simulink model "traffic_blind_test"  (Simulink 8.7)
settings: Solver=FixedStepAuto  StartTime=0.0  StopTime=75  FixedStep=0.01  RelTol=1e-3
settings Model: Creator=eispin  LastModifiedBy=eispin
settings DataIOCC: LimitDataPoints=off  SaveFormat=Dataset
settings DebuggingCC: UnderspecifiedInitializationDetection=Simplified  MergeDetectMultiDrivingBlocksExec=error
settings HardwareCC: ProdBitPerPointer=64  ProdLargestAtomicFloat=Float  ProdIntDivRoundTo=Zero  ProdEndianess=LittleEndian  ProdWordSize=64  ProdHWDeviceType=Intel->x86-64 (Windows64)
settings ModelReferenceCC: PropagateSignalLabelsOutOfModel=on
settings ConfigComp: CovModelRefEnable=off

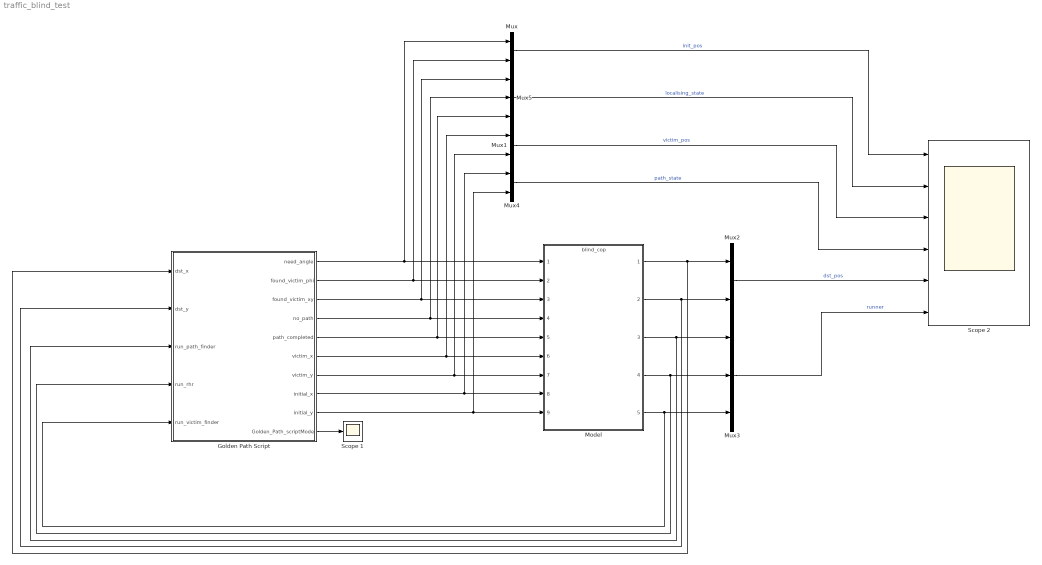
== system traffic_blind_test ==
  Golden Path Script : Stateflow chart  TreatAsAtomicUnit=on
  Model : ModelReference  ModelNameDialog=blind_cop  SimulationMode=Normal  ModelReferenceVersion=1.102
  Mux{,1..2,4} (4 alike) : Mux  Inputs=2
  Mux3 : Mux  Inputs=3
  Mux5 : Mux  Inputs=3
  Scope 1 : Scope
  Scope 2 : Scope  NumInputPorts=6
  wires:
  Model/1 -> Golden Path Script/1(dst_x), Mux2/1
  Model/2 -> Mux2/2, Golden Path Script/2(dst_y)
  Model/3 -> Mux3/1, Golden Path Script/3(run_path_finder)
  Model/4 -> Mux3/2, Golden Path Script/4(run_rhr)
  Model/5 -> Mux3/3, Golden Path Script/5(run_victim_finder)
  Mux3/1 -> Scope 2/6  "runner"
  Mux2/1 -> Scope 2/5  "dst_pos"
  Mux4/1 -> Scope 2/4  "path_state"
  Mux1/1 -> Scope 2/3  "victim_pos"
  Mux5/1 -> Scope 2/2  "localising_state"
  Mux/1 -> Scope 2/1  "init_pos"
  Golden Path Script/1(need_angle) -> Model/1, Mux/1
  Golden Path Script/2(found_victim_phi) -> Model/2, Mux/2
  Golden Path Script/4(no_path) -> Model/4, Mux5/2
  Golden Path Script/3(found_victim_xy) -> Model/3, Mux5/1
  Golden Path Script/6(victim_x) -> Model/6, Mux1/1
  Golden Path Script/5(path_completed) -> Mux5/3, Model/5
  Golden Path Script/7(victim_y) -> Model/7, Mux1/2
  Golden Path Script/8(initial_x) -> Model/8, Mux4/1
  Golden Path Script/9(initial_y) -> Model/9, Mux4/2
  Golden Path Script/10(Golden_Path_scriptMode) -> Scope 1/1

== stateflow chart Golden Path Script ==
  state Consistent
    state InitWait
      en:
      expect_dst_x = -1;
      expect_dst_y = -1;
      expect_run_path_finder = 0;
      expect_run_rhr = 1;
      expect_run_victim_finder = 0;
    state StartInterruptA
      en:
      need_angle = 1;
      expect_run_rhr = 0;
      expect_run_victim_finder = 1;
    state DoneInterruptA
      en:
      need_angle = 0;
    state DoneIsrA
      en:
      found_victim_phi = 1;
      expect_run_victim_finder = 0;
    state resumeAfterA
      en:
      found_victim_phi = 0;
      expect_run_rhr = 1;
    state StartInterruptB
      en:
      need_angle = 1;
      expect_run_rhr = 0;
      expect_run_victim_finder = 1;
    state DoneInterruptB
      en:
      found_victim_phi = 1;
      expect_run_victim_finder = 0;
    state DoneIsrB
      en:
      need_angle = 0;
    state resumeAfterB
      en:
      found_victim_phi = 0;
      expect_run_rhr = 1;
    state DoneIsrC
      en:
      found_victim_xy = 1;
      expect_run_victim_finder = 0;
      expect_run_path_finder = 1;
      expect_dst_x = victim_x;
      expect_dst_y = victim_y;
    state StartInterruptC
      en:
      need_angle = 1;
      expect_run_rhr = 0;
      expect_run_victim_finder = 1;
    state PathFailingA
      % Note that traffic cop should be
      % time-unaware here
      en:
      no_path = 1;
      expect_run_rhr = 1;
      expect_run_path_finder = 0;
    state RhrNearlyOverA
      en:
      expect_run_rhr = -1;
      expect_run_path_finder = -1;
    state RhrOverA
      en:
      % Still expect victim's coords!
      expect_run_rhr = 0;
      expect_run_path_finder = 1;
    state RhringA
      % Check that it doesn't depend on
      % no_path in a weird way
      en:
      no_path = 0;
    state DoneA
      en:
      path_completed = 1;
      expect_run_path_finder = 0;
    state DockingA
      % Waited to make sure that the traffic cop waits on us.
      en:
      path_completed = 0;
      expect_run_path_finder = -1;
      expect_dst_x = -1;
      expect_dst_y = -1;
    state ResumeAfterA
      en:
      expect_run_path_finder = 1;
      expect_dst_x = initial_x;
      expect_dst_y = initial_y;
    state RhrNearlyOverB
      en:
      expect_run_rhr = -1;
      expect_run_path_finder = -1;
    state RhringB
      % Check that it doesn't depend on
      % no_path in a weird way
      en:
      no_path = 0;
    state DoneB
      en:
      path_completed = 1;
      expect_run_path_finder = 0;
    state PathFailingb
      % Note that traffic cop should be
      % time-unaware here
      en:
      no_path = 1;
      expect_run_rhr = 1;
      expect_run_path_finder = 0;
    state RhrOverB
      en:
      % Still expect initial coords!
      expect_run_rhr = 0;
      expect_run_path_finder = 1;
    state TestReaction1
      en:
      path_completed = 0;
    state TestReaction2
      en:
      no_path = 1;
    state TestReaction3
      en:
      found_victim_xy = 1;
    state TestReaction4
      en:
      need_angle = 1;
    state TestReaction5
      en:
      found_victim_phi = 1;
    state TestReaction6
      en:
      path_completed = 1;
    state TestReaction7
      en:
      found_victim_xy = 1;
      initial_x = 12;
      initial_y = 11;
      victim_x = 10;
      victim_y = 9.01;
    state TestReaction8
      en:
      need_angle = 1;
    note: And then, try to confuse the traffic cop by sending random bullshit
        | (which it should ignore)
    (default) -> InitWait
    DoneIsrB -> resumeAfterB : [after(0.5,sec)]
    DoneIsrA -> resumeAfterA : [after(0.5,sec)]
    InitWait -> StartInterruptA : [after(0.5,sec)]
    resumeAfterA -> StartInterruptB : [after(0.5,sec)]
    resumeAfterB -> StartInterruptC : [after(0.5,sec)]
    StartInterruptA -> DoneInterruptA : [after(0.5,sec)]
    StartInterruptB -> DoneInterruptB : [after(0.5,sec)]
    StartInterruptC -> DoneIsrC : [after(0.5,sec)]
    DoneInterruptA -> DoneIsrA : [after(0.5,sec)]
    DoneInterruptB -> DoneIsrB : [after(0.5,sec)]
    DoneIsrC -> PathFailingA : [after(0.5,sec)]
    ResumeAfterA -> PathFailingb : [after(0.5,sec)]
    PathFailingA -> RhringA : [after(0.5,sec)]
    PathFailingb -> RhringB : [after(29,sec)]
    RhringA -> RhrNearlyOverA : [after(29, sec)]
    RhringB -> RhrNearlyOverB : [after(0.5, sec)]
    RhrNearlyOverA -> RhrOverA [order 1] : [is_timeout == 0 && run_path_finder == 1 && run_rhr == 0]
    RhrNearlyOverA -> RhrNearlyOverA [order 2] : [after(1,sec)]{is_timeout = 1;}
    RhrNearlyOverB -> RhrOverB [order 1] : [is_timeout == 0 && run_path_finder == 1 && run_rhr == 0]
    RhrNearlyOverB -> RhrNearlyOverB [order 2] : [after(1,sec)]{is_timeout = 1;}
    RhrOverA -> DoneA : [after(0.5,sec)]
    RhrOverB -> DoneB : [after(0.5,sec)]
    DoneA -> DockingA : [after(0.5,sec)]
    DockingA -> ResumeAfterA [order 2] : [is_timeout==0 && run_path_finder == 1]
    DockingA -> DockingA [order 1] : [after(0.2,sec)]{is_timeout=1;}
    DoneB -> TestReaction1 : [after(0.5,sec)]
    TestReaction3 -> TestReaction6 : [after(0.5,sec)]
    TestReaction6 -> TestReaction5 : [after(0.5,sec)]
    TestReaction1 -> TestReaction2 : [after(0.5,sec)]
    TestReaction5 -> TestReaction8 : [after(0.5,sec)]
    TestReaction2 -> TestReaction4 : [after(0.5,sec)]
    TestReaction8 -> TestReaction7 : [after(0.5,sec)]
    TestReaction4 -> TestReaction3 : [after(0.5,sec)]
  state Failing
    en:
    rem = 2
    du:
    assert(rem > 0);
    rem = rem - 1;
    state bad_x
    state bad_y1
    state bad_r_pf
    state bad_r_rhr
    state bad_r_vf
    state bad_time
    state bad_combo
  note: Note that all "expectations" that are set in "entry" sections
      | will only be checked *next* step, as superstep semantics
      | should be off!
  (default) -> Consistent : {initial_x = 13.37; initial_y = 42;
      |  found_victim_phi = 0; need_angle = 0; found_victim_xy = 0;
      |  victim_x = 3.1416; victim_y = 2.7183;
      |  path_completed = 0; no_path = 0;
      |  expect_dst_x = -1; expect_dst_y = -1;
      |  expect_run_path_finder = -1; expect_run_rhr = -1; expect_run_victim_finder = -1;
      |  is_timeout = 0;}
  Consistent -> bad_x [order 1] : [expect_dst_x >= 0 && dst_x ~= expect_dst_x]
  Consistent -> bad_y1 [order 4] : [expect_dst_y >= 0 && dst_y ~= expect_dst_y]
  Consistent -> bad_r_pf [order 2] : [expect_run_path_finder >= 0 && run_path_finder ~= expect_run_path_finder]
  Consistent -> bad_r_rhr [order 3] : [expect_run_rhr >= 0 && run_rhr ~= expect_run_rhr]
  Consistent -> bad_r_vf [order 5] : [expect_run_victim_finder >= 0 && run_victim_finder ~= expect_run_victim_finder]
  Consistent -> bad_time [order 6] : [is_timeout ~= 0]
  Consistent -> bad_combo [order 7] : [run_path_finder + run_rhr + run_victim_finder > 1]
  data: need_angle output double; found_victim_phi output double; found_victim_xy output double; no_path output double; path_completed output double; victim_x output double; victim_y output double; initial_x output double; initial_y output double; dst_x input double; dst_y input double; run_path_finder input double; run_rhr input double; run_victim_finder input double; expect_dst_x local double; expect_run_rhr local double; expect_run_victim_finder local double; expect_dst_y local double; expect_run_path_finder local double; Golden_Path_scriptMode output Enum: Golden_Path_scriptModeType1; is_timeout local double; rem local double
